simulink library "tqr"  (R2021b)
settings: Solver=VariableStepAuto  StartTime=0.0  StopTime=10.0  RelTol=1e-3
undefined symbols (not defined in the file or in its folder): ATQR_AltRDCActiveREDUInc_X_pct, ATQR_AltRDCActiveREDUInc_Y_enum, ATQR_AltRDCActiveREDUTs_X_pct, ATQR_AltRDCActiveREDUTs_Y_enum, ATQR_CreepREDUTqIncSR_X_rpm, ATQR_CreepREDUTqIncSR_Y_Nm, ATQR_CreepREDUTs_X_rpm, ATQR_CreepREDUTs_Y_Nm, ATQR_EcoTqRrIncGain_X_Nm, ATQR_EcoTqRrIncGain_Y_pct, ATQR_EL1REDUTqDecSR_Y_Nm, ATQR_EL1REDUTqIncSR_X_rpm, ATQR_EL1REDUTqIncSR_Y_pct, ATQR_EL1REDUTs_X_rpm, ATQR_EL1REDUTs_Y_Nm, ATQR_NL1REDUTqDecSR_Y_Nm, ATQR_NL1REDUTqIncSR_X_rpm, ATQR_NL1REDUTqIncSR_Y_pct, ATQR_NL1REDUTs_X_rpm, ATQR_NL1REDUTs_Y_Nm, ATQR_NormalTqRrIncGain_X_Nm, ATQR_NormalTqRrIncGain_Y_pct, ATQR_REDUTIPOutTs_X_rpm, ATQR_RrNegRateLimitIncN_X_rpm, ATQR_RrNegRateLimitIncN_Y_Nm, ATQR_RrPosRateLimitIncN_X_rpm, ATQR_RrPosRateLimitIncN_Y_Nm, ATQR_RTqZeroTransUpBoundN_X_rpm, ATQR_SL1REDUTqDecSR_Y_Nm, ATQR_SL1REDUTqIncSR_X_rpm, ATQR_SL1REDUTqIncSR_Y_pct, ATQR_SL1REDUTs_X_rpm, ATQR_SL1REDUTs_Y_Nm, ATQR_SportTqRrIncGain_X_Nm, ATQR_SportTqRrIncGain_Y_pct, ENUM_CANRDCACTSTA_EXITIMMEDIATELY, ENUM_DRIVEMODE_ECO, ENUM_DRIVEMODE_NRM, ENUM_DRIVEMODE_SPORT, ENUM_GEARACTUALPOSN_R, ENUM_RDCACTSTA_NOREQUEST, ENUM_TQZEROTRANS_NEGATIVE, ENUM_TQZEROTRANS_NOZEROTRANS, ENUM_TQZEROTRANS_POSITIVE, FALSE, KTQD_FrTMTotalGearRatio_gain, KTQD_RrTMTotalGearRatio_gain, KTQR_ARegenLatchEnTq_Nm, KTQR_DriveModeChangeTq_Nm, KTQR_DriveModeCMDTqDev_Nm, KTQR_FinalFEDUTrqLowLim_Nm, KTQR_FinalFEDUTrqUpLim_Nm, KTQR_FinalREDUTrqLowLim_Nm, KTQR_FinalREDUTrqUpLim_Nm, KTQR_FrTMGearEff_c, KTQR_GearEnChangeTq_Nm, KTQR_PreLoadTs_c, KTQR_RrTMGearEff_c, KTQR_TIPOutTsAPS_pct, KTQR_TIPOutTsSpd_kph ... (+44)
libraries: hcu_lib x7, simulink x6
(part 1 of 3)
settings Model: Creator=13615  LastModifiedBy=zack
settings SolverCC: AlgebraicLoopSolver=TrustRegion
settings DataIOCC: SaveFormat=Array  SignalLoggingSaveFormat=ModelDataLogs  ReturnWorkspaceOutputs=off
settings OptimizationCC: BlockReduction=off  BooleanDataType=off
settings DebuggingCC: SaveWithParameterizedLinksMsg=none  UnderspecifiedInitializationDetection=Classic  MergeDetectMultiDrivingBlocksExec=none  SignalResolutionControl=TryResolveAllWithWarning  SFMachineParentedDataDiag=warning
settings HardwareCC: TargetUnknown=on
settings ModelReferenceCC: PropagateSignalLabelsOutOfModel=off
settings ConfigComp: CovMetricSettings=dw  CovSaveCumulativeToWorkspaceVar=on  CovSaveSingleToWorkspaceVar=on

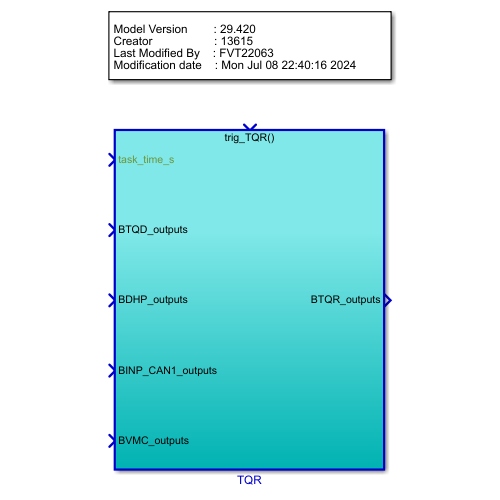
[thumbnail: Simulink's stored preview of the top-level diagram]
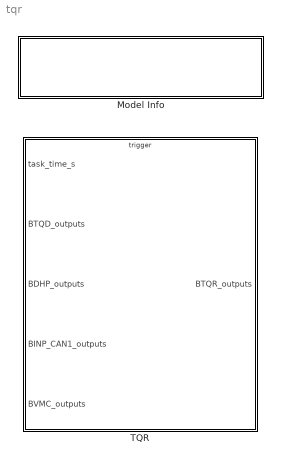
== system tqr ==
  Model Info : Subsystem  LoadFcn=slcm LoadBlock;  InitFcn=slcm('UpdateAllCMBlocksInThisModelInit')  mask(CMBlock){InitialSaveTempField=, InitialBlockCM=None, BlockCM=None, Frame=on, SaveTempField=, DisplayStringWithTags=|, MaskDisplayString=Model Version        : 29.423\nCreator                   : 13615\nLast Modified By    : zack\nModification date    : Tue Jul 16 21:05:23 2024, HorizontalTextAlignment=Left, LeftAlignmentValue=0.02, SourceBlockDiagram=tqr, TagMaxNumber=20, CMTag1=, CMTag2=, CMTag3=, CMTag4=, CMTag5=, CMTag6=, CMTag7=, CMTag8=, CMTag9=, CMTag10=, CMTag11=, CMTag12=, CMTag13=, CMTag14=, CMTag15=, CMTag16=, CMTag17=, CMTag18=, CMTag19=, CMTag20=}
      mask DisplayStringWithTags=|
      | Model Version        : %<ModelVersion>
      | Creator                   : %<Creator>
      | Last Modified By    : %<LastModifiedBy>
      | Modification date    : %<LastModificationDate>
      mask help: This block allows revision control information to be displayed within the model.
      settings: CopyFcn=slcm CopyBlock;  DeleteFcn=slcm Cancel;  PostSaveFcn=slcm('UpdateAllCMBlocksInThisModel')  NameChangeFcn=slcm Rename;  OpenFcn=slcm
      mask Display: text(str2num(LeftAlignmentValue), 0.5, MaskDisplayString, 'HorizontalAlignment', HorizontalTextAlignment)
  TQR : Subsystem  TreatAsAtomicUnit=on
      settings: RTWSystemCode=Nonreusable function  RTWFcnNameOpts=Use subsystem name  RTWFileNameOpts=Use subsystem name

== system tqr/Model Info ==
  EmptySubsystem : Subsystem

== system tqr/TQR ==
  task_time_s : Inport
  BTQD_outputs : Inport  Port=2  OutDataTypeStr=Bus: BTQD_outputs
  BDHP_outputs : Inport  Port=3  OutDataTypeStr=Bus: BDHP_outputs
  BINP_CAN1_outputs : Inport  Port=4  OutDataTypeStr=Bus: BINP_CAN1_outputs
  BVMC_outputs : Inport  Port=5  OutDataTypeStr=Bus: BVMC_outputs
  trig_TQR : TriggerPort  TriggerType=function-call  VariantControl=(inherit)
  Bus Creator : BusCreator  Inputs=9
  Bus Selector : BusSelector  OutputSignals=VINP_FASpeed_kph
  Bus Selector1 : BusSelector  OutputSignals=VTQD_GearActualPosn_enum,VTQD_TqTargetShaftSpd_rpm,VTQD_EVDriveMode_enum,VTQD_AfterAvailableTqDemRr_Nm,VTQD_AfterAvailableTqDemFr_Nm,VTQD_LimpHomeAct_flg,VTQD_PreLoadHold_flg,VTQD_PreLoadPreEn_flg,VTQD_CreepPrLoadEnable_flg,VTQD_RDCActive_enum,VTQD_FrEDUAvailBrkRgnTq_Nm,VTQD_RrEDUAvailBrkRgnTq_Nm,VTQD_RegenMode_enum,VTQD_CoordTqDem_Nm,VTQD_CoordWhlTqDemFr_Nm,VTQD_CoordWhlTqDemRr_Nm,VTQD_FrEDUSpRat_rat,VTQD_RrEDUSpRat_rat
  Bus Selector2 : BusSelector  OutputSignals=VDHP_ActAPSPosn_pct
  Bus Selector5 : BusSelector  OutputSignals=VVMC_ActMaxSlideRate_pct
  Cast To Boolean1 : DataTypeConversion  OutDataTypeStr=boolean
  Cast To Boolean3 : DataTypeConversion  OutDataTypeStr=boolean
  Cast To Boolean4 : DataTypeConversion  OutDataTypeStr=single
  Cast To Boolean5 : DataTypeConversion  OutDataTypeStr=single
  Determine Torque Request : Subsystem
  Ground{2..5} (4 alike) : Ground
  BTQR_outputs : Outport  OutDataTypeStr=Bus: BTQR_outputs
  wires:
  Determine Torque Request/1(VTQR_FrTMTqReq_Nm) -> Bus Creator/1
  Bus Creator/1 -> BTQR_outputs/1  "BTQR_outputs"
  BTQD_outputs/1 -> Bus Selector1/1
  task_time_s/1 -> Determine Torque Request/1(task_time_s)  "task_time_s"
  Determine Torque Request/2(VTQR_FEDUTMSpdReq_rpm) -> Bus Creator/2
  Bus Selector1/1 -> Determine Torque Request/2(VT QD_GearActualPosn_enum)  "<VTQD_GearActualPosn_enum>"
  Bus Selector1/2 -> Determine Torque Request/3(VTQD_TqTargetShaftSpd_rpm)  "<VTQD_TqTargetShaftSpd_rpm>"
  Determine Torque Request/3(VTQR_RrTMTqReq_Nm) -> Bus Creator/3
  Determine Torque Request/4(VTQR_REDUTMSpdReq_rpm) -> Bus Creator/4
  Bus Selector1/3 -> Determine Torque Request/4(<VTQD_EVDriveMode_enum>)  "<VTQD_EVDriveMode_enum>"
  Bus Selector1/4 -> Determine Torque Request/5(<VTQD_AfterAvailableTqDemRr_Nm>)  "<VTQD_AfterAvailableTqDemRr_Nm>"
  Bus Selector1/5 -> Determine Torque Request/6(<VTQD_AfterAvailableTqDemFr_Nm>)  "<VTQD_AfterAvailableTqDemFr_Nm>"
  Bus Selector/1 -> Determine Torque Request/21(VINP_VehSpeed_kph)  "<VINP_FASpeed_kph>"
  Bus Selector1/6 -> Determine Torque Request/7(VTQD_LimpHomeAct_flg)  "<VTQD_LimpHomeAct_flg>"
  BDHP_outputs/1 -> Bus Selector2/1
  Bus Selector2/1 -> Determine Torque Request/20(VDHP_ActAPSPosn_pct)  "<VDHP_ActAPSPosn_pct>"
  Determine Torque Request/6(VTQR_ActualREDUWhlTqReq_Nm) -> Bus Creator/6
  Determine Torque Request/5(VTQR_ActualFEDUWhlTqReq_Nm) -> Bus Creator/5
  BVMC_outputs/1 -> Bus Selector5/1
  Determine Torque Request/7(VTQR_NoABSFEDUWhlTqReq_Nm) -> Bus Creator/7
  Determine Torque Request/8(VTQR_NoABSREDUWhlTqReq_Nm) -> Bus Creator/8
  Bus Selector1/7 -> Determine Torque Request/8(VTQD_PreLoadHold_flg)  "<VTQD_PreLoadHold_flg>"
  Bus Selector1/8 -> Determine Torque Request/9(VTQD_PreLoadPreEn_flg)  "<VTQD_PreLoadPreEn_flg>"
  Bus Selector1/9 -> Determine Torque Request/10(VTQD_CreepPrLoadEnable_flg)  "<VTQD_CreepPrLoadEnable_flg>"
  Bus Selector1/10 -> Determine Torque Request/11(VTQD_RDCActive_enum)  "<VTQD_RDCActive_enum>"
  Bus Selector5/1 -> Determine Torque Request/26(VVMC_ActMaxSlideRate_pct)  "<VVMC_ActMaxSlideRate_pct>"
  BINP_CAN1_outputs/1 -> Bus Selector/1
  Bus Selector1/11 -> Determine Torque Request/12(VTQD_FrEDUAvailBrkRgnTq_Nm)  "<VTQD_FrEDUAvailBrkRgnTq_Nm>"
  Bus Selector1/12 -> Determine Torque Request/13(VTQD_RrEDUAvailBrkRgnTq_Nm)  "<VTQD_RrEDUAvailBrkRgnTq_Nm>"
  Bus Selector1/13 -> Determine Torque Request/14(VTQD_RegenMode_enum)  "<VTQD_RegenMode_enum>"
  Ground2/1 -> Cast To Boolean1/1
  Ground3/1 -> Cast To Boolean3/1
  Ground4/1 -> Cast To Boolean4/1
  Ground5/1 -> Cast To Boolean5/1
  Cast To Boolean1/1 -> Determine Torque Request/22(VINP_FrRBCActive_flg)  "VINP_FrRBCActive_flg"
  Cast To Boolean3/1 -> Determine Torque Request/23(VINP_RrRBCActive_flg)  "VINP_RrRBCActive_flg"
  Cast To Boolean4/1 -> Determine Torque Request/24(VINP_FrntAxlTrqReqBrk_Nm)  "VINP_FrntAxlTrqReqBrk_Nm"
  Cast To Boolean5/1 -> Determine Torque Request/25(VINP_RearAxlTrqReqBrk_Nm)  "VINP_RearAxlTrqReqBrk_Nm"
  Bus Selector1/14 -> Determine Torque Request/15(VTQD_CoordTqDem_Nm)  "<VTQD_CoordTqDem_Nm>"
  Determine Torque Request/9(VTQR_RampREDUWhlTqReq_Nm) -> Bus Creator/9
  Bus Selector1/15 -> Determine Torque Request/16(VTQD_CoordWhlTqDemFr_Nm)  "<VTQD_CoordWhlTqDemFr_Nm>"
  Bus Selector1/16 -> Determine Torque Request/17(VTQD_CoordWhlTqDemRr_Nm)  "<VTQD_CoordWhlTqDemRr_Nm>"
  Bus Selector1/17 -> Determine Torque Request/18(VTQD_FrEDUSpRat_rat)  "<VTQD_FrEDUSpRat_rat>"
  Bus Selector1/18 -> Determine Torque Request/19(VTQD_RrEDUSpRat_rat)  "<VTQD_RrEDUSpRat_rat>"

== system tqr/Model Info/EmptySubsystem ==

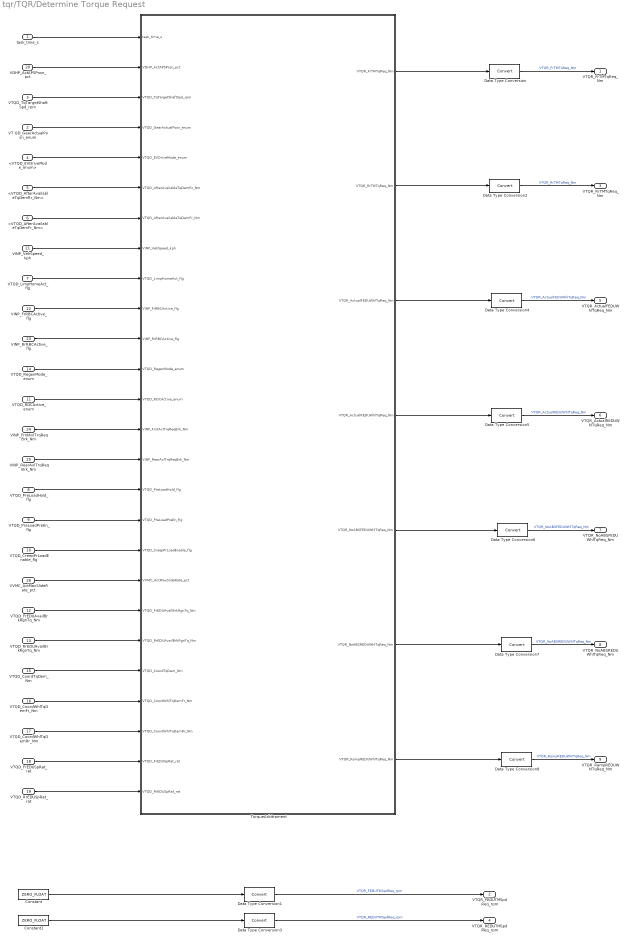
== system tqr/TQR/Determine Torque Request ==
  task_time_s : Inport
  VT QD_GearActualPosn_enum : Inport  Port=2
  VTQD_TqTargetShaftSpd_rpm : Inport  Port=3
  <VTQD_EVDriveMode_enum> : Inport  Port=4
  <VTQD_AfterAvailableTqDemRr_Nm> : Inport  Port=5
  <VTQD_AfterAvailableTqDemFr_Nm> : Inport  Port=6
  VTQD_LimpHomeAct_flg : Inport  Port=7
  VTQD_PreLoadHold_flg : Inport  Port=8
  VTQD_PreLoadPreEn_flg : Inport  Port=9
  VTQD_CreepPrLoadEnable_flg : Inport  Port=10
  VTQD_RDCActive_enum : Inport  Port=11
  VTQD_FrEDUAvailBrkRgnTq_Nm : Inport  Port=12
  VTQD_RrEDUAvailBrkRgnTq_Nm : Inport  Port=13
  VTQD_RegenMode_enum : Inport  Port=14
  VTQD_CoordTqDem_Nm : Inport  Port=15
  VTQD_CoordWhlTqDemFr_Nm : Inport  Port=16
  VTQD_CoordWhlTqDemRr_Nm : Inport  Port=17
  VTQD_FrEDUSpRat_rat : Inport  Port=18
  VTQD_RrEDUSpRat_rat : Inport  Port=19
  VDHP_ActAPSPosn_pct : Inport  Port=20
  VINP_VehSpeed_kph : Inport  Port=21
  VINP_FrRBCActive_flg : Inport  Port=22
  VINP_RrRBCActive_flg : Inport  Port=23
  VINP_FrntAxlTrqReqBrk_Nm : Inport  Port=24
  VINP_RearAxlTrqReqBrk_Nm : Inport  Port=25
  VVMC_ActMaxSlideRate_pct : Inport  Port=26
  Constant : Constant  Value=ZERO_FLOAT  OutDataTypeStr=single
  Constant1 : Constant  Value=ZERO_FLOAT  OutDataTypeStr=single
  Data Type Conversion{,1..8} (9 alike) : DataTypeConversion
  TorqueArbitrament : Subsystem
  VTQR_FrTMTqReq_Nm : Outport
  VTQR_FEDUTMSpdReq_rpm : Outport  Port=2
  VTQR_RrTMTqReq_Nm : Outport  Port=3
  VTQR_REDUTMSpdReq_rpm : Outport  Port=4
  VTQR_ActualFEDUWhlTqReq_Nm : Outport  Port=5
  VTQR_ActualREDUWhlTqReq_Nm : Outport  Port=6
  VTQR_NoABSFEDUWhlTqReq_Nm : Outport  Port=7
  VTQR_NoABSREDUWhlTqReq_Nm : Outport  Port=8
  VTQR_RampREDUWhlTqReq_Nm : Outport  Port=9
  wires:
  TorqueArbitrament/1(VTQR_FrTMTqReq_Nm) -> Data Type Conversion/1
  Constant/1 -> Data Type Conversion1/1
  task_time_s/1 -> TorqueArbitrament/1(task_time_s)
  VT QD_GearActualPosn_enum/1 -> TorqueArbitrament/4(VTQD_GearActualPosn_enum)
  Data Type Conversion/1 -> VTQR_FrTMTqReq_Nm/1  "VTQR_FrTMTqReq_Nm"
  Data Type Conversion1/1 -> VTQR_FEDUTMSpdReq_rpm/1  "VTQR_FEDUTMSpdReq_rpm"
  VTQD_TqTargetShaftSpd_rpm/1 -> TorqueArbitrament/3(VTQD_TqTargetShaftSpd_rpm)
  VDHP_ActAPSPosn_pct/1 -> TorqueArbitrament/2(VDHP_ActAPSPosn_pct)
  TorqueArbitrament/2(VTQR_RrTMTqReq_Nm) -> Data Type Conversion2/1
  Data Type Conversion2/1 -> VTQR_RrTMTqReq_Nm/1  "VTQR_RrTMTqReq_Nm"
  Data Type Conversion3/1 -> VTQR_REDUTMSpdReq_rpm/1  "VTQR_REDUTMSpdReq_rpm"
  Constant1/1 -> Data Type Conversion3/1
  <VTQD_EVDriveMode_enum>/1 -> TorqueArbitrament/5(VTQD_EVDriveMode_enum)
  <VTQD_AfterAvailableTqDemRr_Nm>/1 -> TorqueArbitrament/6(VTQD_AfterAvailableTqDemRr_Nm)
  <VTQD_AfterAvailableTqDemFr_Nm>/1 -> TorqueArbitrament/7(VTQD_AfterAvailableTqDemFr_Nm)
  VINP_VehSpeed_kph/1 -> TorqueArbitrament/8(VINP_VehSpeed_kph)
  VTQD_LimpHomeAct_flg/1 -> TorqueArbitrament/9(VTQD_LimpHomeAct_flg)
  VINP_FrRBCActive_flg/1 -> TorqueArbitrament/10(VINP_FrRBCActive_flg)
  VINP_RrRBCActive_flg/1 -> TorqueArbitrament/11(VINP_RrRBCActive_flg)
  VTQD_RegenMode_enum/1 -> TorqueArbitrament/12(VTQD_RegenMode_enum)
  TorqueArbitrament/3(VTQR_ActualFEDUWhlTqReq_Nm) -> Data Type Conversion4/1
  TorqueArbitrament/4(VTQR_ActualREDUWhlTqReq_Nm) -> Data Type Conversion5/1
  Data Type Conversion4/1 -> VTQR_ActualFEDUWhlTqReq_Nm/1  "VTQR_ActualFEDUWhlTqReq_Nm"
  Data Type Conversion5/1 -> VTQR_ActualREDUWhlTqReq_Nm/1  "VTQR_ActualREDUWhlTqReq_Nm"
  VTQD_RDCActive_enum/1 -> TorqueArbitrament/13(VTQD_RDCActive_enum)
  VINP_FrntAxlTrqReqBrk_Nm/1 -> TorqueArbitrament/14(VINP_FrntAxlTrqReqBrk_Nm)
  VINP_RearAxlTrqReqBrk_Nm/1 -> TorqueArbitrament/15(VINP_RearAxlTrqReqBrk_Nm)
  Data Type Conversion6/1 -> VTQR_NoABSFEDUWhlTqReq_Nm/1  "VTQR_NoABSFEDUWhlTqReq_Nm"
  TorqueArbitrament/6(VTQR_NoABSREDUWhlTqReq_Nm) -> Data Type Conversion7/1
  TorqueArbitrament/5(VTQR_NoABSFEDUWhlTqReq_Nm) -> Data Type Conversion6/1
  VTQD_PreLoadHold_flg/1 -> TorqueArbitrament/16(VTQD_PreLoadHold_flg)
  VTQD_PreLoadPreEn_flg/1 -> TorqueArbitrament/17(VTQD_PreLoadPreEn_flg)
  VTQD_CreepPrLoadEnable_flg/1 -> TorqueArbitrament/18(VTQD_CreepPrLoadEnable_flg)
  Data Type Conversion7/1 -> VTQR_NoABSREDUWhlTqReq_Nm/1  "VTQR_NoABSREDUWhlTqReq_Nm"
  VVMC_ActMaxSlideRate_pct/1 -> TorqueArbitrament/19(VVMC_ActMaxSlideRate_pct)
  VTQD_FrEDUAvailBrkRgnTq_Nm/1 -> TorqueArbitrament/20(VTQD_FrEDUAvailBrkRgnTq_Nm)
  VTQD_RrEDUAvailBrkRgnTq_Nm/1 -> TorqueArbitrament/21(VTQD_RrEDUAvailBrkRgnTq_Nm)
  VTQD_CoordTqDem_Nm/1 -> TorqueArbitrament/22(VTQD_CoordTqDem_Nm)
  TorqueArbitrament/7(VTQR_RampREDUWhlTqReq_Nm) -> Data Type Conversion8/1
  Data Type Conversion8/1 -> VTQR_RampREDUWhlTqReq_Nm/1  "VTQR_RampREDUWhlTqReq_Nm"
  VTQD_CoordWhlTqDemFr_Nm/1 -> TorqueArbitrament/23(VTQD_CoordWhlTqDemFr_Nm)
  VTQD_CoordWhlTqDemRr_Nm/1 -> TorqueArbitrament/24(VTQD_CoordWhlTqDemRr_Nm)
  VTQD_FrEDUSpRat_rat/1 -> TorqueArbitrament/25(VTQD_FrEDUSpRat_rat)
  VTQD_RrEDUSpRat_rat/1 -> TorqueArbitrament/26(VTQD_RrEDUSpRat_rat)

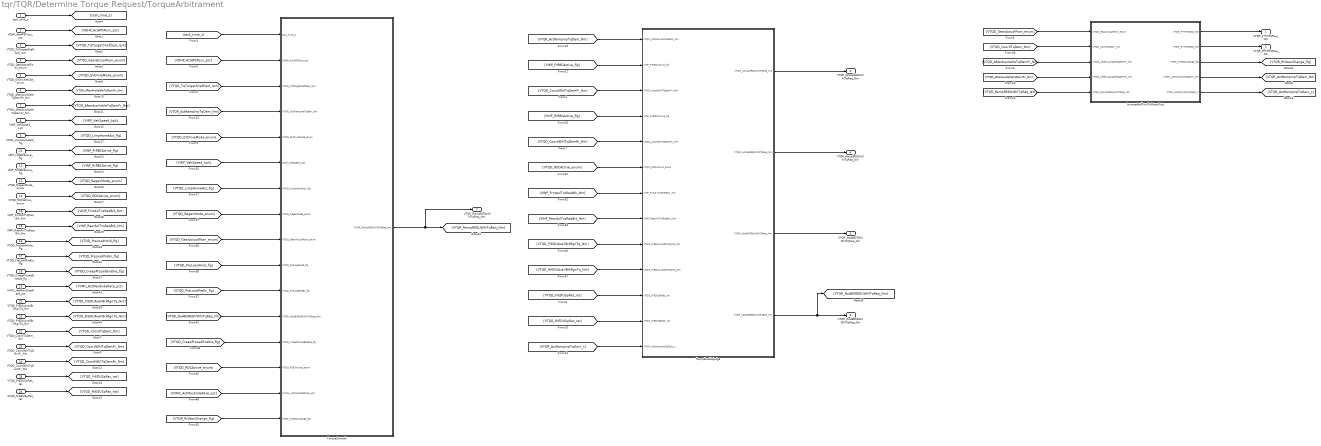
== system tqr/TQR/Determine Torque Request/TorqueArbitrament ==
  task_time_s : Inport
  VDHP_ActAPSPosn_pct : Inport  Port=2
  VTQD_TqTargetShaftSpd_rpm : Inport  Port=3
  VTQD_GearActualPosn_enum : Inport  Port=4
  VTQD_EVDriveMode_enum : Inport  Port=5
  VTQD_AfterAvailableTqDemRr_Nm : Inport  Port=6
  VTQD_AfterAvailableTqDemFr_Nm : Inport  Port=7
  VINP_VehSpeed_kph : Inport  Port=8
  VTQD_LimpHomeAct_flg : Inport  Port=9
  VINP_FrRBCActive_flg : Inport  Port=10
  VINP_RrRBCActive_flg : Inport  Port=11
  VTQD_RegenMode_enum : Inport  Port=12
  VTQD_RDCActive_enum : Inport  Port=13
  VINP_FrntAxlTrqReqBrk_Nm : Inport  Port=14
  VINP_RearAxlTrqReqBrk_Nm : Inport  Port=15
  VTQD_PreLoadHold_flg : Inport  Port=16
  VTQD_PreLoadPreEn_flg : Inport  Port=17
  VTQD_CreepPrLoadEnable_flg : Inport  Port=18
  VVMC_ActMaxSlideRate_pct : Inport  Port=19
  VTQD_FrEDUAvailBrkRgnTq_Nm : Inport  Port=20
  VTQD_RrEDUAvailBrkRgnTq_Nm : Inport  Port=21
  VTQD_CoordTqDem_Nm : Inport  Port=22
  VTQD_CoordWhlTqDemFr_Nm : Inport  Port=23
  VTQD_CoordWhlTqDemRr_Nm : Inport  Port=24
  VTQD_FrEDUSpRat_rat : Inport  Port=25
  VTQD_RrEDUSpRat_rat : Inport  Port=26
  InverseAndTurnToMotorToq : Subsystem
  RampEnableJudge : Subsystem
  TorqueSmooth : Subsystem
  VTQR_FrTMTqReq_Nm : Outport
  VTQR_RrTMTqReq_Nm : Outport  Port=2
  VTQR_ActualFEDUWhlTqReq_Nm : Outport  Port=3
  VTQR_ActualREDUWhlTqReq_Nm : Outport  Port=4
  VTQR_NoABSFEDUWhlTqReq_Nm : Outport  Port=5
  VTQR_NoABSREDUWhlTqReq_Nm : Outport  Port=6
  VTQR_RampREDUWhlTqReq_Nm : Outport  Port=7
  wires:
  task_time_s/1 -> [task_time_s]
  [task_time_s] -> TorqueSmooth/1(task_time_s)
  VTQD_GearActualPosn_enum/1 -> [VTQD_GearActualPosn_enum]
  InverseAndTurnToMotorToq/1(VTQR_FrTMTqReq_Nm) -> VTQR_FrTMTqReq_Nm/1
  [VTQD_GearActualPosn_enum] -> InverseAndTurnToMotorToq/1(VTQD_GearActualPosn_enum)
  VTQD_TqTargetShaftSpd_rpm/1 -> [VTQD_TqTargetShaftSpd_rpm]
  [VTQD_TqTargetShaftSpd_rpm] -> TorqueSmooth/3(VTQD_TqTargetShaftSpd_rpm)
  VDHP_ActAPSPosn_pct/1 -> [VDHP_ActAPSPosn_pct]
  [VDHP_ActAPSPosn_pct] -> TorqueSmooth/2(VDHP_ActAPSPosn_pct)
  InverseAndTurnToMotorToq/2(VTQR_RrTMTqReq_Nm) -> VTQR_RrTMTqReq_Nm/1
  VTQD_EVDriveMode_enum/1 -> [VTQD_EVDriveMode_enum]
  VTQD_AfterAvailableTqDemRr_Nm/1 -> [VTQD_AfterAvailableTqDemRr_Nm]
  VTQD_AfterAvailableTqDemFr_Nm/1 -> [VTQD_AfterAvailableTqDemFr_Nm]
  [VTQD_EVDriveMode_enum] -> TorqueSmooth/5(VTQD_EVDriveMode_enum)
  VINP_VehSpeed_kph/1 -> [VINP_VehSpeed_kph]
  [VINP_VehSpeed_kph] -> TorqueSmooth/6(VINP_VehSpeed_kph)
  VTQD_LimpHomeAct_flg/1 -> [VTQD_LimpHomeAct_flg]
  [VTQD_LimpHomeAct_flg] -> TorqueSmooth/7(VTQD_LimpHomeAct_flg)
  RampEnableJudge/1(VTQR_ActualFEDUWhlTqReq_Nm) -> VTQR_ActualFEDUWhlTqReq_Nm/1
  RampEnableJudge/2(VTQR_ActualREDUWhlTqReq_Nm) -> VTQR_ActualREDUWhlTqReq_Nm/1
  TorqueSmooth/1(VTQR_RampREDUWhlTqReq_Nm) -> VTQR_RampREDUWhlTqReq_Nm/1, [VTQR_RampREDUWhlTqReq_Nm]
  VINP_FrRBCActive_flg/1 -> [VINP_FrRBCActive_flg]
  VINP_RrRBCActive_flg/1 -> [VINP_RrRBCActive_flg]
  [VINP_FrRBCActive_flg] -> RampEnableJudge/2(VINP_FrRBCActive_flg)
  [VINP_RrRBCActive_flg] -> RampEnableJudge/4(VINP_RrRBCActive_flg)
  VTQD_RegenMode_enum/1 -> [VTQD_RegenMode_enum]
  [VTQD_RegenMode_enum] -> TorqueSmooth/8(VTQD_RegenMode_enum)
  VTQD_RDCActive_enum/1 -> [VTQD_RDCActive_enum]
  VINP_FrntAxlTrqReqBrk_Nm/1 -> [VINP_FrntAxlTrqReqBrk_Nm]
  VINP_RearAxlTrqReqBrk_Nm/1 -> [VINP_RearAxlTrqReqBrk_Nm]
  [VTQD_GearActualPosn_enum] -> TorqueSmooth/9(VTQD_GearActualPosn_enum)
  [VTQD_RDCActive_enum] -> RampEnableJudge/6(VTQD_RDCActive_enum)
  [VINP_FrntAxlTrqReqBrk_Nm] -> RampEnableJudge/7(VINP_FrntAxlTrqReqBrk_Nm)
  [VINP_RearAxlTrqReqBrk_Nm] -> RampEnableJudge/8(VINP_RearAxlTrqReqBrk_Nm)
  RampEnableJudge/4(VTQR_NoABSREDUWhlTqReq_Nm) -> [VTQR_NoABSREDUWhlTqReq_Nm], VTQR_NoABSREDUWhlTqReq_Nm/1
  RampEnableJudge/3(VTQR_NoABSFEDUWhlTqReq_Nm) -> VTQR_NoABSFEDUWhlTqReq_Nm/1
  VTQD_PreLoadPreEn_flg/1 -> [VTQD_PreLoadPreEn_flg]
  VTQD_PreLoadHold_flg/1 -> [VTQD_PreLoadHold_flg]
  [VTQD_PreLoadHold_flg] -> TorqueSmooth/10(VTQD_PreLoadHold_flg)
  [VTQD_PreLoadPreEn_flg] -> TorqueSmooth/11(VTQD_PreLoadPreEn_flg)
  [VTQR_NoABSREDUWhlTqReq_Nm] -> TorqueSmooth/12(VTQR_NoABSREDUWhlTqReq_Nm)
  VTQD_CreepPrLoadEnable_flg/1 -> [VTQD_CreepPrLoadEnable_flg]
  [VTQD_CreepPrLoadEnable_flg] -> TorqueSmooth/13(VTQD_CreepPrLoadEnable_flg)
  [VTQD_RDCActive_enum] -> TorqueSmooth/14(VTQD_RDCActive_enum)
  VVMC_ActMaxSlideRate_pct/1 -> [VVMC_ActMaxSlideRate_pct]
  [VVMC_ActMaxSlideRate_pct] -> TorqueSmooth/15(VVMC_ActMaxSlideRate_pct)
  InverseAndTurnToMotorToq/3(VTQR_RrGearChange_flg) -> [VTQR_RrGearChange_flg]
  [VTQR_RrGearChange_flg] -> TorqueSmooth/16(VTQR_RrGearChange_flg)
  [VTQD_FrEDUAvailBrkRgnTq_Nm] -> RampEnableJudge/9(VTQD_FrEDUAvailBrkRgnTq_Nm)
  [VTQD_RrEDUAvailBrkRgnTq_Nm] -> RampEnableJudge/10(VTQD_RrEDUAvailBrkRgnTq_Nm)
  VTQD_FrEDUAvailBrkRgnTq_Nm/1 -> [VTQD_FrEDUAvailBrkRgnTq_Nm]
  VTQD_RrEDUAvailBrkRgnTq_Nm/1 -> [VTQD_RrEDUAvailBrkRgnTq_Nm]
  VTQD_CoordTqDem_Nm/1 -> [VTQD_CoordTqDem_Nm]
  [VTQD_CoordTqDem_Nm] -> InverseAndTurnToMotorToq/2(VTQD_CoordTqDem_Nm)
  InverseAndTurnToMotorToq/4(VTQR_ActRampInpTqDem_Nm) -> [VTQR_ActRampInpTqDem_Nm]
  [VTQR_ActRampInpTqDem_Nm] -> TorqueSmooth/4(VTQR_ActRampInpTqDem_Nm)
  VTQD_CoordWhlTqDemFr_Nm/1 -> [VTQD_CoordWhlTqDemFr_Nm]
  VTQD_CoordWhlTqDemRr_Nm/1 -> [VTQD_CoordWhlTqDemRr_Nm]
  [VTQD_CoordWhlTqDemFr_Nm] -> RampEnableJudge/3(VTQD_CoordWhlTqDemFr_Nm)
  [VTQD_CoordWhlTqDemRr_Nm] -> RampEnableJudge/5(VTQD_CoordWhlTqDemRr_Nm)
  [VTQR_ActRampInpTqDem_Nm] -> RampEnableJudge/1(VTQR_ActRampInpTqDem_Nm)
  VTQD_RrEDUSpRat_rat/1 -> [VTQD_RrEDUSpRat_rat]
  VTQD_FrEDUSpRat_rat/1 -> [VTQD_FrEDUSpRat_rat]
  [VTQD_FrEDUSpRat_rat] -> RampEnableJudge/11(VTQD_FrEDUSpRat_rat)
  [VTQD_RrEDUSpRat_rat] -> RampEnableJudge/12(VTQD_RrEDUSpRat_rat)
  InverseAndTurnToMotorToq/5(VTQR_ActRampInpTqGain_c) -> [VTQR_ActRampInpTqGain_c]
  [VTQR_ActRampInpTqGain_c] -> RampEnableJudge/13(VTQR_ActRampInpTqGain_c)
  [VTQD_AfterAvailableTqDemFr_Nm] -> InverseAndTurnToMotorToq/3(VTQD_AfterAvailableTqDemFr_Nm)
  [VTQD_AfterAvailableTqDemRr_Nm] -> InverseAndTurnToMotorToq/4(VTQD_AfterAvailableTqDemRr_Nm)
  [VTQR_RampREDUWhlTqReq_Nm] -> InverseAndTurnToMotorToq/5(VTQR_RampREDUWhlTqReq_Nm)

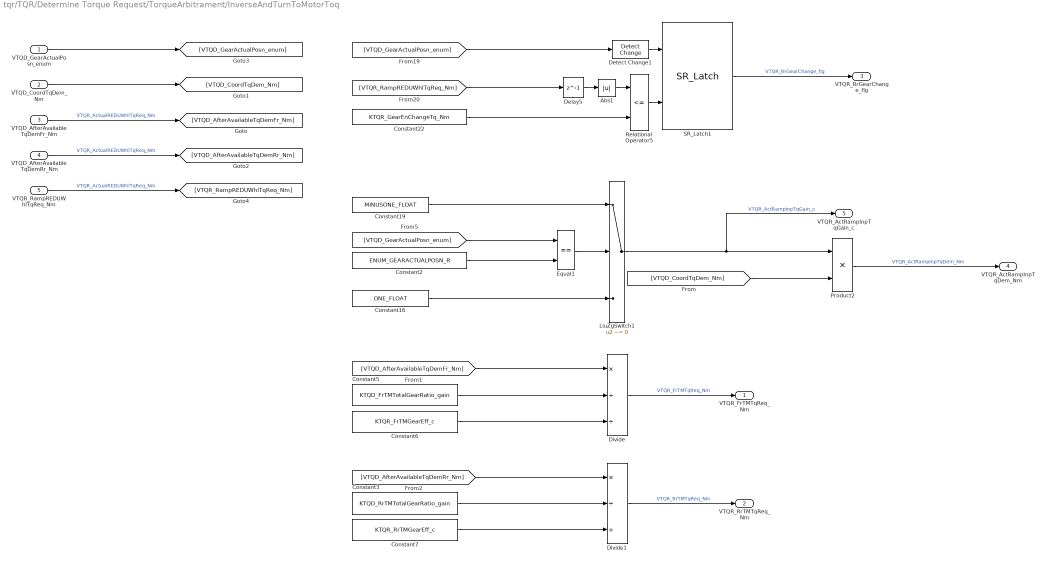
== system tqr/TQR/Determine Torque Request/TorqueArbitrament/InverseAndTurnToMotorToq ==
  VTQD_GearActualPosn_enum : Inport
  VTQD_CoordTqDem_Nm : Inport  Port=2
  VTQD_AfterAvailableTqDemFr_Nm : Inport  Port=3
  VTQD_AfterAvailableTqDemRr_Nm : Inport  Port=4
  VTQR_RampREDUWhlTqReq_Nm : Inport  Port=5
  Abs1 : Abs
  Constant16 : Constant  Value=ONE_FLOAT
  Constant19 : Constant  Value=MINUSONE_FLOAT
  Constant2 : Constant  Value=ENUM_GEARACTUALPOSN_R
  Constant22 : Constant  Value=KTQR_GearEnChangeTq_Nm
  Constant3 : Constant  Value=KTQD_RrTMTotalGearRatio_gain
  Constant5 : Constant  Value=KTQD_FrTMTotalGearRatio_gain
  Constant6 : Constant  Value=KTQR_FrTMGearEff_c
  Constant7 : Constant  Value=KTQR_RrTMGearEff_c
  Delay5 : Delay  DelayLength=1
  Detect Change1 : simulink/Logic and Bit Operations/Detect Change  vinit=0  OutDataTypeStr=boolean
  Divide : Product  Inputs=*//
  Divide1 : Product  Inputs=*//
  Equal1 : RelationalOperator  Operator===  OutDataTypeStr=boolean  RndMeth=Simplest
  LiuZgSwitch1 : Switch  Criteria=u2 ~= 0  Threshold=0.5
      settings: AttributesFormatString=<%<Criteria>>
  Product2 : Product
  Relational Operator5 : RelationalOperator  Operator=<=  OutDataTypeStr=boolean  RndMeth=Simplest
  SR_Latch1 : hcu_lib/Basic_Blocks/SR_Latch
  VTQR_FrTMTqReq_Nm : Outport
  VTQR_RrTMTqReq_Nm : Outport  Port=2
  VTQR_RrGearChange_flg : Outport  Port=3
  VTQR_ActRampInpTqDem_Nm : Outport  Port=4
  VTQR_ActRampInpTqGain_c : Outport  Port=5
  wires:
  Constant6/1 -> Divide/3
  Divide1/1 -> VTQR_RrTMTqReq_Nm/1  "VTQR_RrTMTqReq_Nm"
  Divide/1 -> VTQR_FrTMTqReq_Nm/1  "VTQR_FrTMTqReq_Nm"
  Constant2/1 -> Equal1/2
  Equal1/1 -> LiuZgSwitch1/2
  [VTQD_GearActualPosn_enum] -> Equal1/1
  VTQD_AfterAvailableTqDemFr_Nm/1 -> [VTQD_AfterAvailableTqDemFr_Nm]  "VTQR_ActualREDUWhlTqReq_Nm"
  Constant5/1 -> Divide/2
  Constant3/1 -> Divide1/2
  Constant7/1 -> Divide1/3
  VTQD_GearActualPosn_enum/1 -> [VTQD_GearActualPosn_enum]
  Delay5/1 -> Abs1/1
  Constant22/1 -> Relational Operator5/2
  Abs1/1 -> Relational Operator5/1
  Relational Operator5/1 -> SR_Latch1/2
  SR_Latch1/1 -> VTQR_RrGearChange_flg/1  "VTQR_RrGearChange_flg"
  [VTQD_GearActualPosn_enum] -> Detect Change1/1
  Detect Change1/1 -> SR_Latch1/1
  [VTQR_RampREDUWhlTqReq_Nm] -> Delay5/1
  Constant16/1 -> LiuZgSwitch1/3
  LiuZgSwitch1/1 -> VTQR_ActRampInpTqGain_c/1, Product2/1  "VTQR_ActRampInpTqGain_c"
  Constant19/1 -> LiuZgSwitch1/1
  VTQD_CoordTqDem_Nm/1 -> [VTQD_CoordTqDem_Nm]
  [VTQD_CoordTqDem_Nm] -> Product2/2
  Product2/1 -> VTQR_ActRampInpTqDem_Nm/1  "VTQR_ActRampInpTqDem_Nm"
  VTQD_AfterAvailableTqDemRr_Nm/1 -> [VTQD_AfterAvailableTqDemRr_Nm]  "VTQR_ActualREDUWhlTqReq_Nm"
  [VTQD_AfterAvailableTqDemFr_Nm] -> Divide/1
  [VTQD_AfterAvailableTqDemRr_Nm] -> Divide1/1
  VTQR_RampREDUWhlTqReq_Nm/1 -> [VTQR_RampREDUWhlTqReq_Nm]  "VTQR_ActualREDUWhlTqReq_Nm"

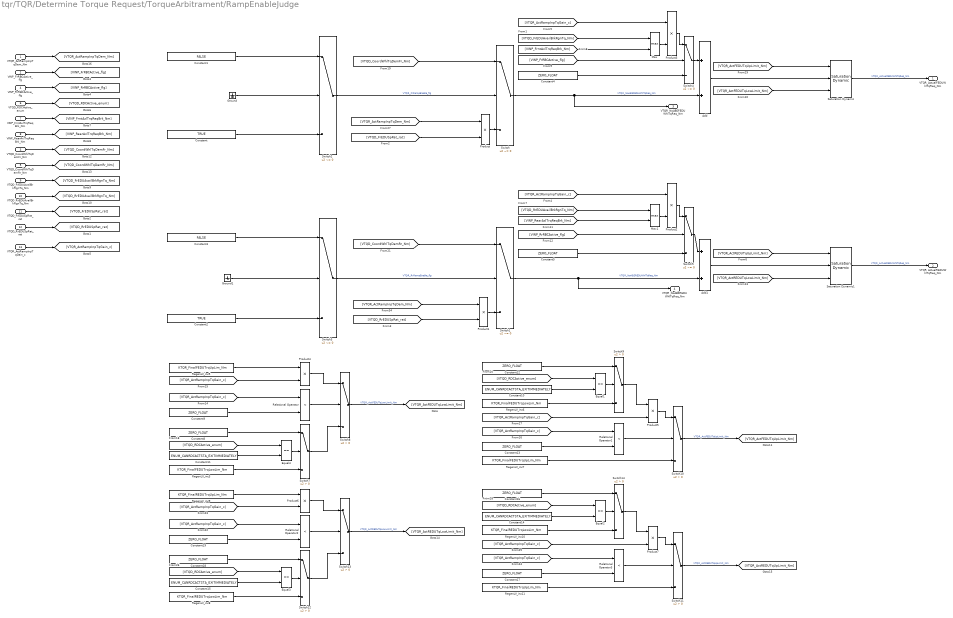
== system tqr/TQR/Determine Torque Request/TorqueArbitrament/RampEnableJudge ==
  VTQR_ActRampInpTqDem_Nm : Inport
  VINP_FrRBCActive_flg : Inport  Port=2
  VTQD_CoordWhlTqDemFr_Nm : Inport  Port=3
  VINP_RrRBCActive_flg : Inport  Port=4
  VTQD_CoordWhlTqDemRr_Nm : Inport  Port=5
  VTQD_RDCActive_enum : Inport  Port=6
  VINP_FrntAxlTrqReqBrk_Nm : Inport  Port=7
  VINP_RearAxlTrqReqBrk_Nm : Inport  Port=8
  VTQD_FrEDUAvailBrkRgnTq_Nm : Inport  Port=9
  VTQD_RrEDUAvailBrkRgnTq_Nm : Inport  Port=10
  VTQD_FrEDUSpRat_rat : Inport  Port=11
  VTQD_RrEDUSpRat_rat : Inport  Port=12
  VTQR_ActRampInpTqGain_c : Inport  Port=13
  Add : Sum
  Add1 : Sum
  Constant : Constant  Value=TRUE
  Constant1 : Constant  Value=FALSE
  Constant{10..11,14..15} (4 alike) : Constant  Value=ENUM_CANRDCACTSTA_EXITIMMEDIATELY
  Constant{4..5,8..9,12..13,16..19} (10 alike) : Constant  Value=ZERO_FLOAT
  Constant2 : Constant  Value=TRUE
  Constant3 : Constant  Value=FALSE
  Equal{1..4} (4 alike) : RelationalOperator  Operator===  OutDataTypeStr=boolean  RndMeth=Simplest
  Ground : Ground
  Ground1 : Ground
  Max : MinMax  Function=max  Inputs=2
  Max1 : MinMax  Function=max  Inputs=2
  Product{,1..7} (8 alike) : Product
  RegenLV_inc10 : Constant  Value=KTQR_FinalREDUTrqLowLim_Nm  OutDataTypeStr=single
  RegenLV_inc11 : Constant  Value=KTQR_FinalREDUTrqUpLim_Nm  OutDataTypeStr=single
  RegenLV_inc3 : Constant  Value=KTQR_FinalFEDUTrqLowLim_Nm  OutDataTypeStr=single
  RegenLV_inc5 : Constant  Value=KTQR_FinalFEDUTrqUpLim_Nm  OutDataTypeStr=single
  RegenLV_inc6 : Constant  Value=KTQR_FinalFEDUTrqLowLim_Nm  OutDataTypeStr=single
  RegenLV_inc7 : Constant  Value=KTQR_FinalFEDUTrqUpLim_Nm  OutDataTypeStr=single
  RegenLV_inc8 : Constant  Value=KTQR_FinalREDUTrqLowLim_Nm  OutDataTypeStr=single
  RegenLV_inc9 : Constant  Value=KTQR_FinalREDUTrqUpLim_Nm  OutDataTypeStr=single
  Relational Operator{,1..3} (4 alike) : RelationalOperator  Operator=<  OutDataTypeStr=boolean  RndMeth=Simplest
  Saturation Dynamic : simulink/Discontinuities/Saturation Dynamic  OutMin=[]  OutMax=[]  OutDataTypeStr=Inherit: Same as second input  OutDataType=fixdt(1, 16)  OutScaling=2^-10  DoSatur=off
  Saturation Dynamic1 : simulink/Discontinuities/Saturation Dynamic  OutMin=[]  OutMax=[]  OutDataTypeStr=Inherit: Same as second input  OutDataType=fixdt(1, 16)  OutScaling=2^-10  DoSatur=off
  Switch{,1..5} (6 alike) : Switch  Criteria=u2 ~= 0
  Switch{7..14} (8 alike) : Switch  Criteria=u2 > Threshold
  VTQR_ActualFEDUWhlTqReq_Nm : Outport
  VTQR_ActualREDUWhlTqReq_Nm : Outport  Port=2
  VTQR_NoABSFEDUWhlTqReq_Nm : Outport  Port=3
  VTQR_NoABSREDUWhlTqReq_Nm : Outport  Port=4
  wires:
  Switch2/1 -> Switch/2  "VTQR_FrRampEnable_flg"
  Switch3/1 -> Switch1/2  "VTQR_RrRampEnable_flg"
  VINP_FrRBCActive_flg/1 -> [VINP_FrRBCActive_flg]
  VINP_RrRBCActive_flg/1 -> [VINP_RrRBCActive_flg]
  VTQD_RDCActive_enum/1 -> [VTQD_RDCActive_enum]
  VINP_FrntAxlTrqReqBrk_Nm/1 -> [VINP_FrntAxlTrqReqBrk_Nm]
  VINP_RearAxlTrqReqBrk_Nm/1 -> [VINP_RearAxlTrqReqBrk_Nm]
  Constant/1 -> Switch2/3
  Constant1/1 -> Switch2/1
  Constant3/1 -> Switch3/1
  Constant2/1 -> Switch3/3
  Switch4/1 -> Add/1
  Constant4/1 -> Switch4/3
  VTQD_CoordWhlTqDemFr_Nm/1 -> [VTQD_CoordWhlTqDemFr_Nm]
  [VTQD_CoordWhlTqDemFr_Nm] -> Switch/1
  VTQD_CoordWhlTqDemRr_Nm/1 -> [VTQD_CoordWhlTqDemRr_Nm]
  [VTQD_CoordWhlTqDemRr_Nm] -> Switch1/1
  [VINP_FrRBCActive_flg] -> Switch4/2
  [VINP_RrRBCActive_flg] -> Switch5/2
  Constant5/1 -> Switch5/3
  Switch5/1 -> Add1/1
  VTQR_ActRampInpTqDem_Nm/1 -> [VTQR_ActRampInpTqDem_Nm]
  Add/1 -> Saturation Dynamic/2
  Saturation Dynamic/1 -> VTQR_ActualFEDUWhlTqReq_Nm/1  "VTQR_ActualFEDUWhlTqReq_Nm"
  Add1/1 -> Saturation Dynamic1/2
  Saturation Dynamic1/1 -> VTQR_ActualREDUWhlTqReq_Nm/1  "VTQR_ActualREDUWhlTqReq_Nm"
  Switch/1 -> VTQR_NoABSFEDUWhlTqReq_Nm/1, Add/2  "VTQR_NoABSFEDUWhlTqReq_Nm"
  Switch1/1 -> Add1/2, VTQR_NoABSREDUWhlTqReq_Nm/1  "VTQR_NoABSREDUWhlTqReq_Nm"
  Constant8/1 -> Switch7/1
  Equal4/1 -> Switch7/2
  [VTQD_RDCActive_enum] -> Equal4/1
  Constant11/1 -> Equal4/2
  RegenLV_inc3/1 -> Switch7/3
  [VINP_RearAxlTrqReqBrk_Nm] -> Max1/2
  VTQD_FrEDUAvailBrkRgnTq_Nm/1 -> [VTQD_FrEDUAvailBrkRgnTq_Nm]
  VTQD_RrEDUAvailBrkRgnTq_Nm/1 -> [VTQD_RrEDUAvailBrkRgnTq_Nm]
  [VTQD_RrEDUAvailBrkRgnTq_Nm] -> Max1/1
  [VTQD_FrEDUAvailBrkRgnTq_Nm] -> Max/1
  [VINP_FrntAxlTrqReqBrk_Nm] -> Max/2
  Ground/1 -> Switch2/2
  Ground1/1 -> Switch3/2
  VTQD_RrEDUSpRat_rat/1 -> [VTQD_RrEDUSpRat_rat]
  VTQD_FrEDUSpRat_rat/1 -> [VTQD_FrEDUSpRat_rat]
  Product/1 -> Switch/3
  [VTQD_FrEDUSpRat_rat] -> Product/2
  [VTQR_ActRampInpTqDem_Nm] -> Product/1
  Product1/1 -> Switch1/3
  [VTQR_ActRampInpTqDem_Nm] -> Product1/1
  [VTQD_RrEDUSpRat_rat] -> Product1/2
  Max1/1 -> Product2/2
  Product2/1 -> Switch5/1
  VTQR_ActRampInpTqGain_c/1 -> [VTQR_ActRampInpTqGain_c]
  [VTQR_ActRampInpTqGain_c] -> Product2/1
  [VTQR_ActRampInpTqGain_c] -> Product3/1
  Max/1 -> Product3/2
  Product3/1 -> Switch4/1
  Switch7/1 -> Switch8/3
  Relational Operator/1 -> Switch8/2
  [VTQR_ActRampInpTqGain_c] -> Relational Operator/1
  Constant9/1 -> Relational Operator/2
  Switch8/1 -> [VTQR_ActFEDUTqLowLimit_Nm]  "VTQR_ActFEDUTqLowLimit_Nm"
  Product4/1 -> Switch8/1
  RegenLV_inc5/1 -> Product4/1
  [VTQR_ActRampInpTqGain_c] -> Product4/2
  [VTQR_ActREDUTqLowLimit_Nm] -> Saturation Dynamic1/3
  RegenLV_inc6/1 -> Switch9/3
  Constant10/1 -> Equal1/2
  Equal1/1 -> Switch9/2
  Constant13/1 -> Relational Operator1/2
  RegenLV_inc7/1 -> Switch10/3
  Constant12/1 -> Switch9/1
  [VTQR_ActRampInpTqGain_c] -> Relational Operator1/1
  [VTQD_RDCActive_enum] -> Equal1/1
  Relational Operator1/1 -> Switch10/2
  [VTQR_ActRampInpTqGain_c] -> Product5/2
  Product5/1 -> Switch10/1
  Switch9/1 -> Product5/1
  Switch10/1 -> [VTQR_ActFEDUTqUpLimit_Nm]  "VTQR_ActFEDUTqUpLimit_Nm"
  [VTQR_ActREDUTqUpLimit_Nm] -> Saturation Dynamic1/1
  Switch12/1 -> Switch13/3
  Switch11/1 -> [VTQR_ActREDUTqUpLimit_Nm]  "VTQR_ActREDUTqUpLimit_Nm"
  RegenLV_inc8/1 -> Switch12/3
  [VTQR_ActRampInpTqGain_c] -> Product6/2
  Constant15/1 -> Equal3/2
  Constant18/1 -> Switch12/1
  [VTQD_RDCActive_enum] -> Equal3/1
  [VTQR_ActRampInpTqGain_c] -> Product7/2
  RegenLV_inc11/1 -> Switch11/3
  [VTQD_RDCActive_enum] -> Equal2/1
  [VTQR_ActRampInpTqGain_c] -> Relational Operator3/1
  Constant17/1 -> Relational Operator3/2
  Constant16/1 -> Switch14/1
  Equal3/1 -> Switch12/2
  Equal2/1 -> Switch14/2
  Constant14/1 -> Equal2/2
  RegenLV_inc10/1 -> Switch14/3
  Product6/1 -> Switch13/1
  Switch14/1 -> Product7/1
  Product7/1 -> Switch11/1
  Switch13/1 -> [VTQR_ActREDUTqLowLimit_Nm]  "VTQR_ActREDUTqLowLimit_Nm"
  Relational Operator2/1 -> Switch13/2
  Relational Operator3/1 -> Switch11/2
  Constant19/1 -> Relational Operator2/2
  RegenLV_inc9/1 -> Product6/1
  [VTQR_ActRampInpTqGain_c] -> Relational Operator2/1
  [VTQR_ActFEDUTqLowLimit_Nm] -> Saturation Dynamic/3
  [VTQR_ActFEDUTqUpLimit_Nm] -> Saturation Dynamic/1

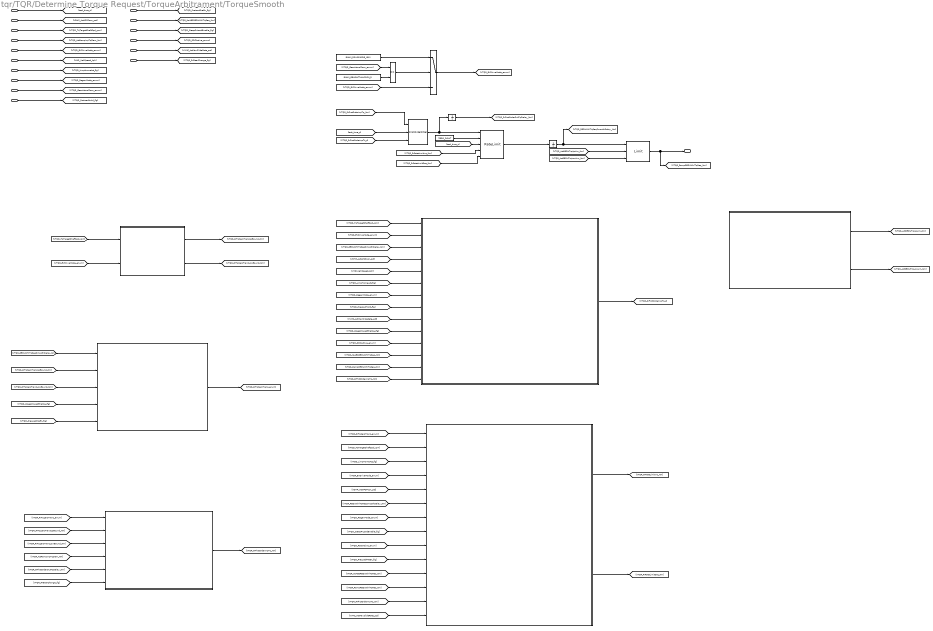
== system tqr/TQR/Determine Torque Request/TorqueArbitrament/TorqueSmooth ==
  note: Rear Rate limitation map and determination
  note: Rear wheel first order filter input torque command determination
  note: Rear Torque zero point transfer status determination
  note: Rear Torque zero point transfer boundary map
  note: Rear First order filter input tau map and determination
  note: Rear torque ramp limtation and determination
  task_time_s : Inport
  VDHP_ActAPSPosn_pct : Inport  Port=2
  VTQD_TqTargetShaftSpd_rpm : Inport  Port=3
  VTQR_ActRampInpTqDem_Nm : Inport  Port=4
  VTQD_EVDriveMode_enum : Inport  Port=5
  VINP_VehSpeed_kph : Inport  Port=6
  VTQD_LimpHomeAct_flg : Inport  Port=7
  VTQD_RegenMode_enum : Inport  Port=8
  VTQD_GearActualPosn_enum : Inport  Port=9
  VTQD_PreLoadHold_flg : Inport  Port=10
  VTQD_PreLoadPreEn_flg : Inport  Port=11
  VTQR_NoABSREDUWhlTqReq_Nm : Inport  Port=12
  VTQD_CreepPrLoadEnable_flg : Inport  Port=13
  VTQD_RDCActive_enum : Inport  Port=14
  VVMC_ActMaxSlideRate_pct : Inport  Port=15
  VTQR_RrGearChange_flg : Inport  Port=16
  Constant1 : Constant  Value=ZERO_FLOAT
  Equal : RelationalOperator  Operator===  OutDataTypeStr=boolean  RndMeth=Simplest
  FirstOrderFilter : hcu_lib/Basic_Blocks/FirstOrderFilter
  Limit : hcu_lib/Basic_Blocks/Limit
  RateLimit1 : hcu_lib/Basic_Blocks/RateLimit
  Rear First order filter input tau map and determination : Subsystem
  Rear Torque zero point transfer boundary map : Subsystem
  "Rear Torque zero point transfer status determination " : Subsystem
  Rear torque ramp limtation and determination : Subsystem
  Rear wheel first order filter input torque command determination : Subsystem
  Rear wheel rate limit determination : Subsystem
  RegenLV_inc5 : Constant  Value=ENUM_GEARACTUALPOSN_R
  RegenLV_inc6 : Constant  Value=ENUM_DRIVEMODE_NRM
  Switch : Switch  Criteria=u2 ~= 0
  Unit Delay2 : UnitDelay  SampleTime=-1
  Unit Delay4 : UnitDelay  SampleTime=-1
  VTQR_RampREDUWhlTqReq_Nm : Outport
  wires:
  task_time_s/1 -> [task_time_s]
  VDHP_ActAPSPosn_pct/1 -> [VDHP_ActAPSPosn_pct]
  VTQR_ActRampInpTqDem_Nm/1 -> [VTQR_ActRampInpTqDem_Nm]
  Unit Delay2/1 -> Limit/1, [VTQR_REDUWhlTqReqSmoothDelay_Nm]  "VTQR_REDUWhlTqReqSmoothDelay_Nm"
  RateLimit1/1 -> Unit Delay2/1  "VTQR_REDUWhlTqReqSmooth_Nm"
  FirstOrderFilter/1 -> RateLimit1/1, Unit Delay4/1  "VTQR_RrFirstOrderOutTq_Nm"
  [task_time_s] -> FirstOrderFilter/2
  Limit/1 -> [VTQR_RampREDUWhlTqReq_Nm], VTQR_RampREDUWhlTqReq_Nm/1  "VTQR_RampREDUWhlTqReq_Nm"
  [task_time_s] -> RateLimit1/3
  Constant1/1 -> RateLimit1/2
  VTQD_EVDriveMode_enum/1 -> [VTQD_EVDriveMode_enum]
  VINP_VehSpeed_kph/1 -> [VINP_VehSpeed_kph]
  VTQD_LimpHomeAct_flg/1 -> [VTQD_LimpHomeAct_flg]
  [VTQR_REDUWhlTqReqSmoothDelay_Nm] -> "Rear Torque zero point transfer status determination "/1(VTQR_REDUWhlTqReqSmoothDelay_Nm)
  [VTQR_RrTqZeroTransUpBound_Nm] -> "Rear Torque zero point transfer status determination "/2(VTQR_RrTqZeroTransUpBound_Nm)
  [VTQR_RrTqZeroTransLowBound_Nm] -> "Rear Torque zero point transfer status determination "/3(VTQR_RrTqZeroTransLowBound_Nm)
  "Rear Torque zero point transfer status determination "/1(VTQR_RrTqZeroTrans_enum) -> [VTQR_RrTqZeroTrans_enum]
  [VTQR_RrTqZeroTrans_enum] -> Rear wheel first order filter input torque command determination/1(VTQR_RrTqZeroTrans_enum)
  [VTQR_RrTqZeroTransUpBound_Nm] -> Rear wheel first order filter input torque command determination/2(VTQR_RrTqZeroTransUpBound_Nm)
  [VTQR_RrTqZeroTransLowBound_Nm] -> Rear wheel first order filter input torque command determination/3(VTQR_RrTqZeroTransLowBound_Nm)
  [VTQR_ActRampInpTqDem_Nm] -> Rear wheel first order filter input torque command determination/4(VTQR_ActRampInpTqDem_Nm)
  [VTQR_RrFirstOrderOutTqDelay_Nm] -> Rear wheel first order filter input torque command determination/5(VTQR_RrFirstOrderOutTqDelay_Nm)
  Rear wheel first order filter input torque command determination/1(VTQR_RrFirstOrderInpTq_Nm) -> [VTQR_RrFirstOrderInpTq_Nm]
  [VTQR_RrFirstOrderInpTq_Nm] -> FirstOrderFilter/1
  Rear wheel rate limit determination/1(VTQR_RrRateLimitInc_Nm) -> [VTQR_RrRateLimitInc_Nm]
  Rear wheel rate limit determination/2(VTQR_RrRateLimitDec_Nm) -> [VTQR_RrRateLimitDec_Nm]
  [VTQD_TqTargetShaftSpd_rpm] -> Rear wheel rate limit determination/2(VTQD_TqTargetShaftSpd_rpm)
  [VTQR_RrTqZeroTrans_enum] -> Rear wheel rate limit determination/1(VTQR_RrTqZeroTrans_enum)
  [VTQR_RrRateLimitInc_Nm] -> RateLimit1/4
  [VTQR_RrRateLimitDec_Nm] -> RateLimit1/5
  Rear First order filter input tau map and determination/1(VTQR_RrFirstOrderInpTs_c) -> [VTQR_RrFirstOrderInpTs_c]
  [VTQR_RrFirstOrderInpTs_c] -> FirstOrderFilter/3
  Unit Delay4/1 -> [VTQR_RrFirstOrderOutTqDelay_Nm]  "VTQR_RrFirstOrderOutTqDelay_Nm"
  [VTQD_TqTargetShaftSpd_rpm] -> Rear First order filter input tau map and determination/1(VTQD_TqTargetShaftSpd_rpm)
  [VTQR_EVDriveMode_enum] -> Rear First order filter input tau map and determination/2(VTQR_EVDriveMode_enum)
  [VTQR_REDUWhlTqReqSmoothDelay_Nm] -> Rear First order filter input tau map and determination/3(VTQR_REDUWhlTqReqSmooth_Nm)
  [VDHP_ActAPSPosn_pct] -> Rear First order filter input tau map and determination/4(VDHP_ActAPSPosn_pct)
  [VINP_VehSpeed_kph] -> Rear First order filter input tau map and determination/5(VINP_VehSpeed_kph)
  [VTQD_LimpHomeAct_flg] -> Rear First order filter input tau map and determination/6(VTQD_LimpHomeAct_flg)
  [VTQD_LimpHomeAct_flg] -> Rear wheel rate limit determination/3(VTQD_LimpHomeAct_flg)
  [VTQR_EVDriveMode_enum] -> Rear wheel rate limit determination/4(VTQR_EVDriveMode_enum)
  [VDHP_ActAPSPosn_pct] -> Rear wheel rate limit determination/5(VDHP_ActAPSPosn_pct)
  [VTQR_REDUWhlTqReqSmoothDelay_Nm] -> Rear wheel rate limit determination/6(VTQR_REDUWhlTqReqSmoothDelay_Nm)
  [VTQD_TqTargetShaftSpd_rpm] -> Rear Torque zero point transfer boundary map/1(VTQD_TqTargetShaftSpd_rpm)
  [VTQR_EVDriveMode_enum] -> Rear Torque zero point transfer boundary map/2(VTQR_EVDriveMode_enum)
  Rear Torque zero point transfer boundary map/1(VTQR_RrTqZeroTransUpBound_Nm) -> [VTQR_RrTqZeroTransUpBound_Nm]
  Rear Torque zero point transfer boundary map/2(VTQR_RrTqZeroTransLowBound_Nm) -> [VTQR_RrTqZeroTransLowBound_Nm]
  VTQD_RegenMode_enum/1 -> [VTQD_RegenMode_enum]
  [VTQD_RegenMode_enum] -> Rear First order filter input tau map and determination/7(VTQD_RegenMode_enum)
  [VTQD_RegenMode_enum] -> Rear wheel rate limit determination/7(VTQD_RegenMode_enum)
  RegenLV_inc5/1 -> Equal/2
  Equal/1 -> Switch/2
  RegenLV_inc6/1 -> Switch/1
  Switch/1 -> [VTQR_EVDriveMode_enum]  "VTQR_EVDriveMode_enum"
  [VTQD_GearActualPosn_enum] -> Equal/1
  [VTQD_EVDriveMode_enum] -> Switch/3
  VTQD_GearActualPosn_enum/1 -> [VTQD_GearActualPosn_enum]
  VTQD_TqTargetShaftSpd_rpm/1 -> [VTQD_TqTargetShaftSpd_rpm]
  VTQD_PreLoadHold_flg/1 -> [VTQD_PreLoadHold_flg]
  VTQD_PreLoadPreEn_flg/1 -> [VTQD_PreLoadPreEn_flg]
  [VTQD_PreLoadHold_flg] -> Rear First order filter input tau map and determination/8(VTQD_PreLoadHold_flg)
  VTQR_NoABSREDUWhlTqReq_Nm/1 -> [VTQR_NoABSREDUWhlTqReq_Nm]
  VTQD_CreepPrLoadEnable_flg/1 -> [VTQD_CreepPrLoadEnable_flg]
  [VTQD_CreepPrLoadEnable_flg] -> "Rear Torque zero point transfer status determination "/4(VTQD_CreepPrLoadEnable_flg)
  [VTQD_PreLoadPreEn_flg] -> "Rear Torque zero point transfer status determination "/5(VTQD_PreLoadPreEn_flg)
  [VTQD_CreepPrLoadEnable_flg] -> Rear First order filter input tau map and determination/10(VTQD_CreepPrLoadEnable_flg)
  VTQD_RDCActive_enum/1 -> [VTQD_RDCActive_enum]
  [VTQD_PreLoadPreEn_flg] -> Rear wheel rate limit determination/10(VTQD_PreLoadPreEn_flg)
  [VTQD_CreepPrLoadEnable_flg] -> Rear wheel rate limit determination/8(VTQD_CreepPrLoadEnable_flg)
  [VTQD_RDCActive_enum] -> Rear wheel rate limit determination/9(VTQD_RDCActive_enum)
  [VTQD_RDCActive_enum] -> Rear First order filter input tau map and determination/11(VTQD_RDCActive_enum)
  [VTQR_NoABSREDUWhlTqReq_Nm] -> Rear First order filter input tau map and determination/12(VTQR_NoABSREDUWhlTqReq_Nm)
  [VTQR_RampREDUWhlTqReq_Nm] -> Rear First order filter input tau map and determination/13(VTQR_RampREDUWhlTqReq_Nm)
  [VTQR_NoABSREDUWhlTqReq_Nm] -> Rear wheel rate limit determination/11(VTQR_NoABSREDUWhlTqReq_Nm)
  [VTQR_RampREDUWhlTqReq_Nm] -> Rear wheel rate limit determination/12(VTQR_RampREDUWhlTqReq_Nm)
  [VTQR_RrFirstOrderInpTq_Nm] -> Rear First order filter input tau map and determination/14(VTQR_RrFirstOrderInpTq_Nm)
  [VTQR_RrFirstOrderInpTq_Nm] -> Rear wheel rate limit determination/13(VTQR_RrFirstOrderInpTq_Nm)
  Rear torque ramp limtation and determination/1(VTQR_ActREDUTrqUpLim_Nm) -> [VTQR_ActREDUTrqUpLim_Nm]
  Rear torque ramp limtation and determination/2(VTQR_ActREDUTrqLowLim_Nm) -> [VTQR_ActREDUTrqLowLim_Nm]
  [VTQR_ActREDUTrqUpLim_Nm] -> Limit/2
  [VTQR_ActREDUTrqLowLim_Nm] -> Limit/3
  VVMC_ActMaxSlideRate_pct/1 -> [VVMC_ActMaxSlideRate_pct]
  [VVMC_ActMaxSlideRate_pct] -> Rear wheel rate limit determination/14(VVMC_ActMaxSlideRate_pct)
  [VVMC_ActMaxSlideRate_pct] -> Rear First order filter input tau map and determination/9(VVMC_ActMaxSlideRate_pct)
  VTQR_RrGearChange_flg/1 -> [VTQR_RrGearChange_flg]
  [VTQR_RrGearChange_flg] -> Rear wheel first order filter input torque command determination/6(VTQR_RrGearChange_flg)

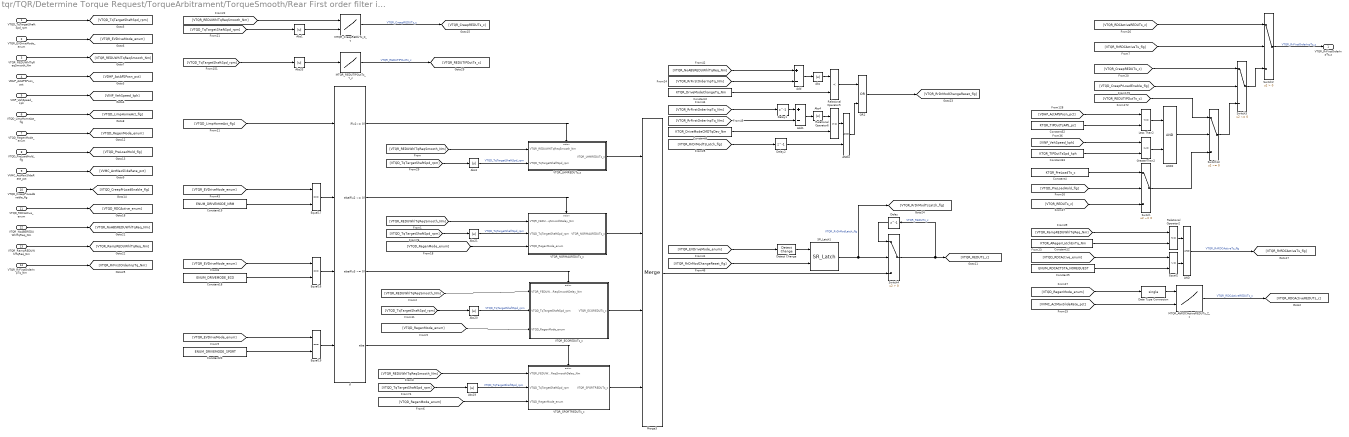
== system tqr/TQR/Determine Torque Request/TorqueArbitrament/TorqueSmooth/Rear First order filter input tau map and determination ==
  VTQD_TqTargetShaftSpd_rpm : Inport
  VTQR_EVDriveMode_enum : Inport  Port=2
  VTQR_REDUWhlTqReqSmooth_Nm : Inport  Port=3
  VDHP_ActAPSPosn_pct : Inport  Port=4
  VINP_VehSpeed_kph : Inport  Port=5
  VTQD_LimpHomeAct_flg : Inport  Port=6
  VTQD_RegenMode_enum : Inport  Port=7
  VTQD_PreLoadHold_flg : Inport  Port=8
  VVMC_ActMaxSlideRate_pct : Inport  Port=9
  VTQD_CreepPrLoadEnable_flg : Inport  Port=10
  VTQD_RDCActive_enum : Inport  Port=11
  VTQR_NoABSREDUWhlTqReq_Nm : Inport  Port=12
  VTQR_RampREDUWhlTqReq_Nm : Inport  Port=13
  VTQR_RrFirstOrderInpTq_Nm : Inport  Port=14
  AND : Logic  AllPortsSameDT=off  OutDataTypeStr=boolean
  AND2 : Logic  AllPortsSameDT=off  OutDataTypeStr=boolean
  AND4 : Logic  AllPortsSameDT=off  OutDataTypeStr=boolean
  Abs{,1,3..4,19..21,33} (8 alike) : Abs
  Add : Sum  Inputs=+-
  Add1 : Sum  Inputs=+-
  Constant12 : Constant  Value=KTQR_ARegenLatchEnTq_Nm
  Constant18 : Constant  Value=ENUM_DRIVEMODE_ECO
  Constant19 : Constant  Value=ENUM_DRIVEMODE_NRM
  Constant2 : Constant  Value=KTQR_DriveModeChangeTq_Nm
  Constant20 : Constant  Value=ENUM_DRIVEMODE_SPORT
  Constant32 : Constant  Value=KTQR_TIPOutTsAPS_pct
  Constant33 : Constant  Value=KTQR_TIPOutTsSpd_kph
  Constant4 : Constant  Value=KTQR_PreLoadTs_c
  Constant5 : Constant  Value=ENUM_RDCACTSTA_NOREQUEST
  Constant8 : Constant  Value=KTQR_DriveModeCMDTqDev_Nm
  Data Type Conversion : DataTypeConversion  OutDataTypeStr=single
  Delay : Delay  DelayLength=1
  Delay1 : Delay  DelayLength=1
  Delay2 : Delay  DelayLength=1
  Detect Change : simulink/Logic and Bit Operations/Detect Change  vinit=0  OutDataTypeStr=boolean
  Equal16 : RelationalOperator  Operator===  OutDataTypeStr=boolean  RndMeth=Simplest
  Equal17 : RelationalOperator  Operator===  OutDataTypeStr=boolean  RndMeth=Simplest
  Equal19 : RelationalOperator  Operator===  OutDataTypeStr=boolean  RndMeth=Simplest
  Equal2 : RelationalOperator  Operator=~=  OutDataTypeStr=boolean  RndMeth=Simplest
  GreaterThan2 : RelationalOperator  OutDataTypeStr=boolean  RndMeth=Simplest
  If : If  NumInputs=4  IfExpression=u1~= 0  ElseIfExpressions=u2 ~= 0, u3 ~= 0
  Less Than2 : RelationalOperator  Operator=<=  OutDataTypeStr=boolean  RndMeth=Simplest
  MTQR_AltRDCActiveREDUTs_Z_c : Lookup_n-D  BreakpointsForDimension1=ATQR_AltRDCActiveREDUTs_Y_enum  BreakpointsForDimension2=ATQR_AltRDCActiveREDUTs_X_pct  Table=MTQR_AltRDCActiveREDUTs_Z_c  TableDataTypeStr=Inherit: Inherit from 'Table data'  ExtrapMethod=Clip  InternalRulePriority=Speed  RndMeth=Simplest  InputSameDT=on
      settings: InputPortMap=u0,u1
  MTQR_CreepREDUTs_Z_c : Lookup_n-D  BreakpointsForDimension1=ATQR_CreepREDUTs_Y_Nm  BreakpointsForDimension2=ATQR_CreepREDUTs_X_rpm  Table=MTQR_CreepREDUTs_Z_c  ExtrapMethod=Clip  InternalRulePriority=Speed  RndMeth=Simplest  InputSameDT=on
      settings: InputPortMap=u0,u1
  MTQR_REDUTIPOutTs_Y_c : Lookup_n-D  NumberOfTableDimensions=1  BreakpointsForDimension1=ATQR_REDUTIPOutTs_X_rpm  Table=MTQR_REDUTIPOutTs_Y_c  ExtrapMethod=Clip  InternalRulePriority=Speed  RndMeth=Simplest  InputSameDT=on
  Merge3 : Merge  Inputs=4
  OR2 : Logic  Operator=OR  AllPortsSameDT=off  OutDataTypeStr=boolean
  Relational Operator2 : RelationalOperator  Operator=<=  OutDataTypeStr=boolean  RndMeth=Simplest
  Relational Operator5 : RelationalOperator  Operator=<  OutDataTypeStr=boolean  RndMeth=Simplest
  Relational Operator6 : RelationalOperator  OutDataTypeStr=boolean  RndMeth=Simplest
  SR_Latch1 : hcu_lib/Basic_Blocks/SR_Latch
  Switch : Switch  Criteria=u2 ~= 0
  Switch13 : Switch  Criteria=u2 ~= 0
  Switch2 : Switch  Criteria=u2 > Threshold
  Switch3 : Switch  Criteria=u2 ~= 0  Threshold=0.5
  Switch4 : Switch  Criteria=u2 > Threshold
  VTQR_ECOREDUTs_c : Subsystem  AncestorBlock=tqr/TQR/Determine Torque Request/TorqueArbitrament/TorqueSmooth/Front First order filter input tau map and determination/VTQR_ECOFEDUTs_c  TreatAsAtomicUnit=on
  VTQR_LHMREDUTs_c : Subsystem  AncestorBlock=tqr/TQR/Determine Torque Request/TorqueArbitrament/TorqueSmooth/VTQR_LHMREDUTs_c  TreatAsAtomicUnit=on
  VTQR_NORMALREDUTs_c : Subsystem  AncestorBlock=tqr/TQR/Determine Torque Request/TorqueArbitrament/TorqueSmooth/Front First order filter input tau map and determination/VTQR_NORMALFEDUTs_c  TreatAsAtomicUnit=on
  VTQR_SPORTREDUTs_c : Subsystem  AncestorBlock=tqr/TQR/Determine Torque Request/TorqueArbitrament/TorqueSmooth/Front First order filter input tau map and determination/VTQR_SPORTFEDUTs_c  TreatAsAtomicUnit=on
  VTQR_RrFirstOrderInpTs_c : Outport
  wires:
  Abs3/1 -> VTQR_LHMREDUTs_c/2(VTQD_TqTargetShaftSpd_rpm)  "VTQD_TqTargetShaftSpd_rpm"
  VTQR_LHMREDUTs_c/1(VTQR_LHMREDUTs_c) -> Merge3/1
  Equal19/1 -> If/4
  Constant18/1 -> Equal16/2
  Constant19/1 -> Equal17/2
  [VTQD_LimpHomeAct_flg] -> If/1
  Equal16/1 -> If/3
  Equal17/1 -> If/2
  [VTQD_TqTargetShaftSpd_rpm] -> Abs3/1
  [VTQR_EVDriveMode_enum] -> Equal16/1
  Constant20/1 -> Equal19/2
  VTQR_NORMALREDUTs_c/1(VTQR_NORMALREDUTs_c) -> Merge3/2
  [VTQR_EVDriveMode_enum] -> Equal19/1
  If/4 -> VTQR_SPORTREDUTs_c/Action
  [VTQR_EVDriveMode_enum] -> Equal17/1
  [VTQD_TqTargetShaftSpd_rpm] -> Abs21/1
  [VTQD_TqTargetShaftSpd_rpm] -> Abs20/1
  [VTQR_REDUWhlTqReqSmooth_Nm] -> VTQR_LHMREDUTs_c/1(VTQR_REDUWhlTqReqSmooth_Nm)
  [VTQD_TqTargetShaftSpd_rpm] -> Abs19/1
  Abs21/1 -> VTQR_NORMALREDUTs_c/2(VTQD_TqTargetShaftSpd_rpm)  "VTQD_TqTargetShaftSpd_rpm"
  If/1 -> VTQR_LHMREDUTs_c/Action
  [VTQR_REDUWhlTqReqSmooth_Nm] -> VTQR_ECOREDUTs_c/1(VTQR_FEDUWhlTqReqSmoothDelay_Nm)
  Abs20/1 -> VTQR_ECOREDUTs_c/2(VTQD_TqTargetShaftSpd_rpm)  "VTQD_TqTargetShaftSpd_rpm"
  [VTQR_REDUWhlTqReqSmooth_Nm] -> VTQR_NORMALREDUTs_c/1(VTQR_FEDUWhlTqReqSmoothDelay_Nm)
  VTQR_SPORTREDUTs_c/1(VTQR_SPORTREDUTs_c) -> Merge3/4
  VTQR_ECOREDUTs_c/1(VTQR_ECOREDUTs_c) -> Merge3/3
  [VTQD_TqTargetShaftSpd_rpm] -> Abs33/1
  Abs33/1 -> MTQR_REDUTIPOutTs_Y_c/1
  MTQR_REDUTIPOutTs_Y_c/1 -> [VTQR_REDUTIPOutTs_c]  "VTQR_REDUTIPOutTs_c"
  VTQR_EVDriveMode_enum/1 -> [VTQR_EVDriveMode_enum]
  VTQD_TqTargetShaftSpd_rpm/1 -> [VTQD_TqTargetShaftSpd_rpm]
  VTQR_REDUWhlTqReqSmooth_Nm/1 -> [VTQR_REDUWhlTqReqSmooth_Nm]
  VTQD_LimpHomeAct_flg/1 -> [VTQD_LimpHomeAct_flg]
  VDHP_ActAPSPosn_pct/1 -> [VDHP_ActAPSPosn_pct]
  VINP_VehSpeed_kph/1 -> [VINP_VehSpeed_kph]
  [VTQD_RegenMode_enum] -> VTQR_NORMALREDUTs_c/3(VTQD_RegenMode_enum)
  [VTQD_RegenMode_enum] -> VTQR_ECOREDUTs_c/3(VTQD_RegenMode_enum)
  [VTQD_RegenMode_enum] -> VTQR_SPORTREDUTs_c/3(VTQD_RegenMode_enum)
  [VTQR_REDUWhlTqReqSmooth_Nm] -> VTQR_SPORTREDUTs_c/1(VTQR_FEDUWhlTqReqSmoothDelay_Nm)
  Abs19/1 -> VTQR_SPORTREDUTs_c/2(VTQD_TqTargetShaftSpd_rpm)  "VTQD_TqTargetShaftSpd_rpm"
  If/3 -> VTQR_ECOREDUTs_c/Action
  If/2 -> VTQR_NORMALREDUTs_c/Action
  VTQD_RegenMode_enum/1 -> [VTQD_RegenMode_enum]
  [VINP_VehSpeed_kph] -> GreaterThan2/1
  Less Than2/1 -> AND2/1
  [VTQR_REDUTIPOutTs_c] -> Switch13/1
  [VTQD_CreepPrLoadEnable_flg] -> Switch3/2
  Switch13/1 -> Switch3/3
  Constant33/1 -> GreaterThan2/2
  GreaterThan2/1 -> AND2/2
  AND2/1 -> Switch13/2
  [VDHP_ActAPSPosn_pct] -> Less Than2/1
  Constant32/1 -> Less Than2/2
  Switch2/1 -> VTQR_RrFirstOrderInpTs_c/1  "VTQR_RrFirstOrderInpTs_c"
  [VTQD_PreLoadHold_flg] -> Switch/2
  Constant4/1 -> Switch/1
  [VTQR_REDUTs_c] -> Switch/3
  Switch/1 -> Switch13/3
  VTQD_PreLoadHold_flg/1 -> [VTQD_PreLoadHold_flg]
  [VTQR_CreepREDUTs_c] -> Switch3/1
  VTQD_CreepPrLoadEnable_flg/1 -> [VTQD_CreepPrLoadEnable_flg]
  Abs1/1 -> MTQR_CreepREDUTs_Z_c/2
  [VTQR_REDUWhlTqReqSmooth_Nm] -> MTQR_CreepREDUTs_Z_c/1
  [VTQD_TqTargetShaftSpd_rpm] -> Abs1/1
  MTQR_CreepREDUTs_Z_c/1 -> [VTQR_CreepREDUTs_c]  "VTQR_CreepREDUTs_c"
  Constant12/1 -> Relational Operator2/2
  [VTQR_RampREDUWhlTqReq_Nm] -> Relational Operator2/1
  [VTQD_RDCActive_enum] -> Equal2/1
  Equal2/1 -> AND/2
  Constant5/1 -> Equal2/2
  AND/1 -> [VTQR_RrRDCActiveTs_flg]  "VTQR_RrRDCActiveTs_flg"
  Relational Operator2/1 -> AND/1
  [VTQR_RrRDCActiveTs_flg] -> Switch2/2
  Switch3/1 -> Switch2/3
  VTQD_RDCActive_enum/1 -> [VTQD_RDCActive_enum]
  VTQR_NoABSREDUWhlTqReq_Nm/1 -> [VTQR_NoABSREDUWhlTqReq_Nm]
  VTQR_RampREDUWhlTqReq_Nm/1 -> [VTQR_RampREDUWhlTqReq_Nm]
  Add/1 -> Abs/1
  Delay2/1 -> AND4/2
  AND4/1 -> OR2/2
  [VTQR_EVDriveMode_enum] -> Detect Change/1
  Constant2/1 -> Relational Operator5/2
  Delay/1 -> Switch4/1
  Switch4/1 -> [VTQR_REDUTs_c], Delay/1  "VTQR_REDUTs_c"
  Relational Operator6/1 -> AND4/1
  Merge3/1 -> Switch4/3
  SR_Latch1/1 -> Switch4/2, [VTQR_RrDrModTsLatch_flg]  "VTQR_RrDrModLatch_flg"
  Delay1/1 -> Add1/1
  Abs/1 -> Relational Operator5/1
  [VTQR_RrDrModChangeReset_flg] -> SR_Latch1/2
  [VTQR_RrDrModTsLatch_flg] -> Delay2/1
  Detect Change/1 -> SR_Latch1/1
  Constant8/1 -> Relational Operator6/2
  Abs4/1 -> Relational Operator6/1
  OR2/1 -> [VTQR_RrDrModChangeReset_flg]
  Add1/1 -> Abs4/1
  [VTQR_RrFirstOrderInpTq_Nm] -> Delay1/1
  [VTQR_RrFirstOrderInpTq_Nm] -> Add1/2
  [VTQR_RrFirstOrderInpTq_Nm] -> Add/2
  Relational Operator5/1 -> OR2/1
  [VTQR_NoABSREDUWhlTqReq_Nm] -> Add/1
  VTQR_RrFirstOrderInpTq_Nm/1 -> [VTQR_RrFirstOrderInpTq_Nm]
  Data Type Conversion/1 -> MTQR_AltRDCActiveREDUTs_Z_c/1
  MTQR_AltRDCActiveREDUTs_Z_c/1 -> [VTQR_RDCActiveREDUTs_c]  "VTQR_RDCActiveREDUTs_c"
  [VTQD_RegenMode_enum] -> Data Type Conversion/1
  [VTQR_RDCActiveREDUTs_c] -> Switch2/1
  VVMC_ActMaxSlideRate_pct/1 -> [VVMC_ActMaxSlideRate_pct]
  [VVMC_ActMaxSlideRate_pct] -> MTQR_AltRDCActiveREDUTs_Z_c/2
